simulink model "nonlinear_sensor"  (R2015a)
settings: Solver=ode3  StartTime=0.0  StopTime=25  FixedStep=0.0001  RelTol=1e-3
libraries: simulink x1
settings Model: Creator=morten  LastModifiedBy=morten

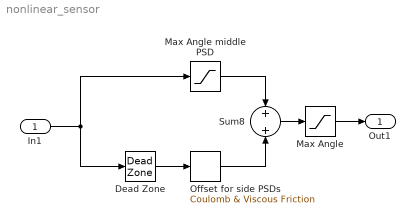
== system nonlinear_sensor ==
  In1 : Inport
  Dead Zone : DeadZone  LowerValue=-0.3225  UpperValue=0.337  SaturateOnIntegerOverflow=on
  Max Angle : Saturate  UpperLimit=0.664  LowerLimit=-0.68
  Max Angle middle PSD : Saturate  UpperLimit=.1627  LowerLimit=-0.1787
  Offset for side PSDs : simulink/Discontinuities/Coulomb & Viscous Friction  offset=[0.225]  gain=1
  Sum8 : Sum  Inputs=+|+
  Out1 : Outport
  wires:
  In1/1 -> Dead Zone/1, Max Angle middle PSD/1
  Sum8/1 -> Max Angle/1
  Max Angle middle PSD/1 -> Sum8/1
  Max Angle/1 -> Out1/1
  Dead Zone/1 -> Offset for side PSDs/1
  Offset for side PSDs/1 -> Sum8/2
